simulink library "speedgoatlib_evse"  (R2024b)
settings: Solver=VariableStepAuto  StartTime=0.0  StopTime=10.0  RelTol=1e-3
undefined symbols (not defined in the file): sg_ev_charging_read_m, sg_ev_charging_write_m, sg_ev_isolation_read_m, sg_ev_parameter_read_m, sg_ev_parameter_write_m, sg_ev_precharge_read_m, sg_ev_precharge_write_m, sg_ev_status_m, sg_ev_stop_read_m, sg_ev_stop_write_m, sg_ev_welding_read_m, sg_ev_welding_write_m, sg_evse_charging_read_m, sg_evse_charging_write_m, sg_evse_isolation_read_m, sg_evse_isolation_write_m, sg_evse_parameter_read_m, sg_evse_parameter_write_m, sg_evse_precharge_read_m, sg_evse_precharge_write_m, sg_evse_status_m, sg_evse_stop_read_m, sg_evse_stop_write_m, sg_evse_welding_read_m, sg_evse_welding_write_m
libraries: speedgoatlib_mqtt x199, simulink x39, $bdroot x24
(part 8 of 8)

== matlab function speedgoatlib_evse/Blocks by Charge State/EVSE Setup /Enabled Subsystem/to physical value format ==
  data: multiplier output; input input; value output
function [multiplier, value] = fcn(input)
    [multiplier, value] = sg_evse.lib_m.toJsonPhysicalValue(input);
end

== matlab function speedgoatlib_evse/Blocks by Charge State/EVSE Setup /Enabled Subsystem/to physical value format1 ==
  data: multiplier output; input input; value output
function [multiplier, value] = fcn(input)
    [multiplier, value] = sg_evse.lib_m.toJsonPhysicalValue(input);
end

== matlab function speedgoatlib_evse/Blocks by Charge State/EVSE Setup /Enabled Subsystem/to physical value format2 ==
  data: multiplier output; input input; value output
function [multiplier, value] = fcn(input)
    [multiplier, value] = sg_evse.lib_m.toJsonPhysicalValue(input);
end

== matlab function speedgoatlib_evse/Blocks by Charge State/EVSE Setup /Enabled Subsystem/to physical value format3 ==
  data: multiplier output; input input; value output
function [multiplier, value] = fcn(input)
    [multiplier, value] = sg_evse.lib_m.toJsonPhysicalValue(input);
end

== matlab function speedgoatlib_evse/Blocks by Charge State/EV Charging Write /Enabled Subsystem/to physical value format ==
  data: multiplier output; input input; value output
function [multiplier, value] = fcn(input)
    [multiplier, value] = sg_evse.lib_m.toJsonPhysicalValue(input);
end
